simulink model "calefaccion_control_prueba_MODIFICADO_Jesus"  (R2021a)
settings: Solver=VariableStepAuto  StartTime=0.0  StopTime=3600*24*15  RelTol=1e-3
values from neighbouring files (symbols this model uses):
  Tref = 16.5    [izaro.m]
libraries: pid_lib x1
settings Model: Creator=izaro.garro  LastModifiedBy=djoroya
settings SolverCC: AlgebraicLoopSolver=TrustRegion
settings DebuggingCC: SFMachineParentedDataDiag=warning
settings SFSimCC: CustomCodeUndefinedFunction=UseInterfaceOnly

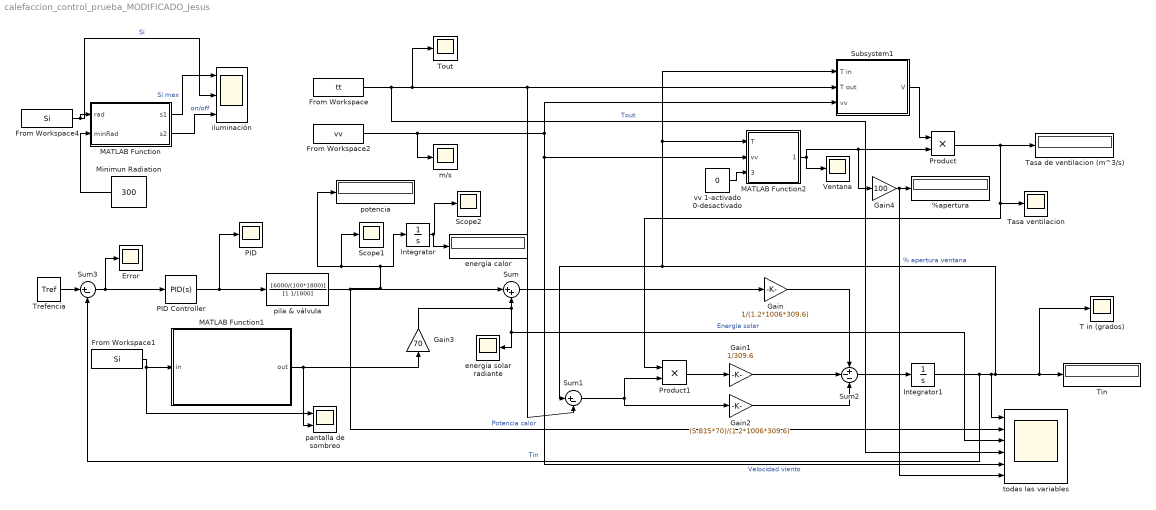
== system calefaccion_control_prueba_MODIFICADO_Jesus ==
  %apertura : Display
  Error : Scope
  From Workspace : FromWorkspace  VariableName=tt  SampleTime=600  ZeroCross=off
  From Workspace1 : FromWorkspace  VariableName=Si  SampleTime=600  ZeroCross=off
  From Workspace2 : FromWorkspace  VariableName=vv  SampleTime=600  ZeroCross=off
  From Workspace4 : FromWorkspace  VariableName=Si  SampleTime=600  ZeroCross=off
  Gain : Gain  Gain=1/(1.2*1006*309.6)
  Gain1 : Gain  Gain=1/309.6
  Gain2 : Gain  Gain=(5.815*70)/(1.2*1006*309.6)
  Gain3 : Gain  Gain=70
  Gain4 : Gain  Gain=100
  Integrator : Integrator
  Integrator1 : Integrator  InitialCondition=20
  MATLAB Function : MATLAB Function  TreatAsAtomicUnit=on  SystemSampleTime=600
  MATLAB Function1 : MATLAB Function  TreatAsAtomicUnit=on  SystemSampleTime=600
  MATLAB Function2 : MATLAB Function  TreatAsAtomicUnit=on  SystemSampleTime=1
  Minimun Radiation : Constant  Value=300
  PID : Scope
  PID Controller : pid_lib/PID Controller  Controller=PID  Form=Parallel  TimeDomain=Continuous-time  UseExternalTs=off  SampleTime=-1  IntegratorMethod=Forward Euler  FilterMethod=Forward Euler  ControllerParametersSource=internal  P=2  I=2/1200  D=0  UseFilter=on  N=0.0006  TunerSelectOption=Transfer Function Based (PID Tuner App)  ZeroCross=off  InitialConditionSource=internal  InitialConditionForIntegrator=0  InitialConditionForFilter=0  DifferentiatorICPrevScaledInput=0  ExternalReset=none  TrackingMode=off  Kt=1  LimitOutput=on  SatLimitsSource=internal  UpperSaturationLimit=100  LowerSaturationLimit=0  LinearizeAsGain=on  AntiWindupMode=clamping  Kb=1  POutMin=[]  POutMax=[]  IOutMin=[]  IOutMax=[]  DOutMin=[]  DOutMax=[]  NOutMin=[]  NOutMax=[]  SumOutMin=[]  SumOutMax=[]  SaturationOutMin=[]  SaturationOutMax=[]  PParamMin=[]  PParamMax=[]  IParamMin=[]  IParamMax=[]  DParamMin=[]  DParamMax=[]  NParamMin=[]  NParamMax=[]  KbParamMin=[]  KbParamMax=[]  KtParamMin=[]  KtParamMax=[]  KbOutMin=[]  KbOutMax=[]  KtOutMin=[]  KtOutMax=[]  IntegratorOutMin=[]  IntegratorOutMax=[]  FilterOutMin=[]  FilterOutMax=[]  SumI1OutMin=[]  SumI1OutMax=[]  SumI2OutMin=[]  SumI2OutMax=[]  SumI3OutMin=[]  SumI3OutMax=[]  SumI4OutMin=[]  SumI4OutMax=[]  SumDOutMin=[]  SumDOutMax=[]  DifferentiatorOutMin=[]  DifferentiatorOutMax=[]  FilterDiffOutCoefMin=[]  FilterDiffOutCoefMax=[]  ReciprocalOutMin=[]  ReciprocalOutMax=[]  SumDenOutMin=[]  SumDenOutMax=[]  SumNumOutMin=[]  SumNumOutMax=[]  DivideOutMin=[]  DivideOutMax=[]  UdiffTsProdOutMin=[]  UdiffTsProdOutMax=[]  NTsProdOutMin=[]  NTsProdOutMax=[]  UintegralTsProdOutMin=[]  UintegralTsProdOutMax=[]  UngainTsProdOutMin=[]  UngainTsProdOutMax=[]  IntegratorContinuousStateAttributes=''  IntegratorStateMustResolveToSignalObject=off  IntegratorRTWStateStorageClass=Auto  FilterContinuousStateAttributes=''  FilterStateMustResolveToSignalObject=off  FilterRTWStateStorageClass=Auto  ParallelPVariant=InternalParameters  IdealPVariant=Disabled  IVariant=InternalParameters  DVariant=InternalParameters  IntegratorVariant=Continuous  SatVariant=Enabled  AWVariant=ContClampingParallel  PCopyVariant=Disabled  TRVariant=Disabled  FdbkBlocksVariant=Forward  IdealPFdbkVariant=Disabled  SatFdbkVariant=Disabled  DerivativeFilterVariant=ContFilter  NVariant=InternalParameters  NCopyVariant=Disabled  FilterICVariant=InternalICsFilter  IntegratorICVariant=InternalICs  ExternalResetVariant=Disabled  TRSumVariant=Passthrough  SumFdbkVariant=Disabled  SumVariant=Sum_PID  TsampFilterVariant=InternalTs  TsampNgainVariant=Passthrough  TsampIntegralVariant=Passthrough  ExternalSaturationOutDataTypeStr=Inherit: Same as second input
  Product : Product
  Product1 : Product
  Scope1 : Scope
  Scope2 : Scope
  Subsystem1 : Subsystem
      mask Display: image('$imagefile'); % Use "Edit Image" on toolstrip to change.
  Sum : Sum  Inputs=|++
  Sum1 : Sum  Inputs=|+-
  Sum2 : Sum  Inputs=+--
  Sum3 : Sum  Inputs=|+-
  T in (grados) : Scope
  Tasa de ventilacion (m^3/s) : Display
  Tasa ventilacion : Scope
  Tin : Display
  Tout : Scope
  Trefencia : Constant  Value=Tref
  Ventana : Scope
  energía calor : Display
  energía solar radiante : Scope
  iluminación : Scope  NumInputPorts=3
  m/s : Scope
  pantalla de sombreo : Scope  NumInputPorts=2
  pila & válvula : TransferFcn  Numerator=[6000/(100*1800)]  Denominator=[1 1/1800]
  potencia : Display
  todas las variables : Scope  NumInputPorts=6
  vv 1-activado 0-desactivado : Constant  Value=0
  wires:
  Sum/1 -> Gain/1
  Gain/1 -> Sum2/1
  Gain1/1 -> Sum2/2
  Product1/1 -> Gain1/1
  Sum1/1 -> Gain2/1, Product1/2
  Gain2/1 -> Sum2/3
  Subsystem1/1(V) -> Product/1
  Sum3/1 -> Error/1, PID Controller/1
  PID Controller/1 -> PID/1, pila & válvula/1
  Trefencia/1 -> Sum3/1
  From Workspace/1 -> todas las variables/4, Tout/1, Sum1/2, Subsystem1/2(T out)  "Tout"
  pila & válvula/1 -> todas las variables/2, Sum/1, Integrator/1, potencia/1, Scope1/1  "Potencia calor"
  Integrator1/1 -> Sum3/2, todas las variables/1, T in (grados)/1, Tin/1, Sum1/1, MATLAB Function2/1(T), Subsystem1/1(T in)  "Tin"
  Gain3/1 -> todas las variables/3, energía solar radiante/1, Sum/2  "Energía solar"
  From Workspace4/1 -> iluminación/2, MATLAB Function/1(rad)  "Si"
  MATLAB Function/1(s1) -> iluminación/1  "Si max"
  MATLAB Function/2(s2) -> iluminación/3  "on/off"
  From Workspace2/1 -> Subsystem1/3(vv), todas las variables/5, MATLAB Function2/2(vv), m/s/1  "Velocidad viento"
  MATLAB Function1/1(out) -> Gain3/1, pantalla de sombreo/2
  From Workspace1/1 -> MATLAB Function1/1(in), pantalla de sombreo/1
  Product/1 -> Tasa de ventilacion (m^3/s)/1, Tasa ventilacion/1, Product1/1
  MATLAB Function2/1(posicionNueva) -> Ventana/1, Gain4/1, Product/2
  Gain4/1 -> todas las variables/6, %apertura/1  "% apertura ventana"
  vv 1-activado 0-desactivado/1 -> MATLAB Function2/3(vv_opcion)
  Integrator/1 -> Scope2/1, energía calor/1
  Sum2/1 -> Integrator1/1
  Minimun Radiation/1 -> MATLAB Function/2(minRad)

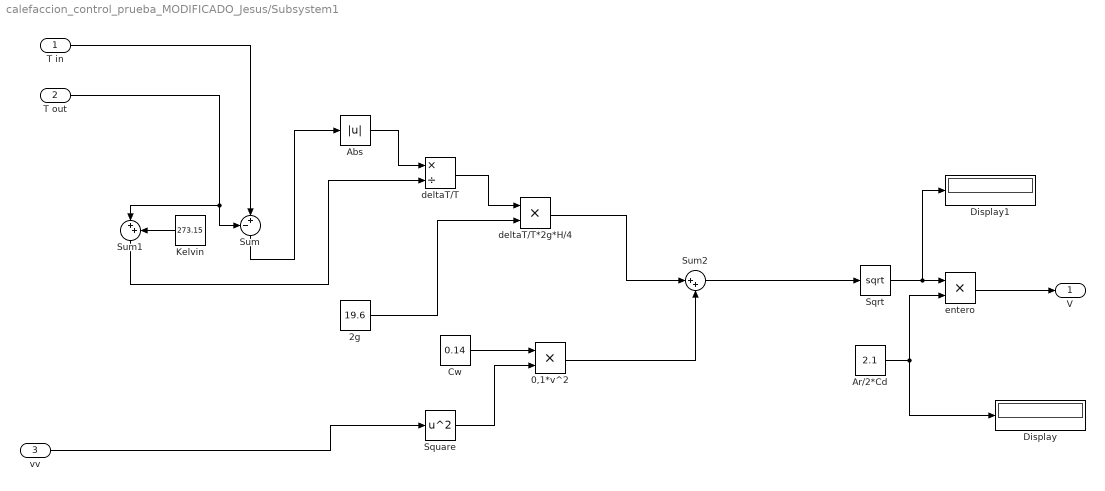
== system calefaccion_control_prueba_MODIFICADO_Jesus/Subsystem1 ==
  T in : Inport
  T out : Inport  Port=2
  vv : Inport  Port=3
  0,1*v^2 : Product  Inputs=**
  2g : Constant  Value=19.6
  Abs : Abs
  Ar/2*Cd : Constant  Value=2.1
  Cw : Constant  Value=0.14
  Display : Display
  Display1 : Display
  Kelvin : Constant  Value=273.15
  Sqrt : Sqrt  SaturateOnIntegerOverflow=on
  Square : Math  Operator=square  SignedPower=on  SaturateOnIntegerOverflow=on
  Sum : Sum  Inputs=-+|
  Sum1 : Sum  Inputs=|++
  Sum2 : Sum  Inputs=|++
  deltaT/T : Product  Inputs=*/
  deltaT/T*2g*H/4 : Product  Inputs=**
  entero : Product  Inputs=**
  V : Outport
  wires:
  T in/1 -> Sum/2
  Sum2/1 -> Sqrt/1
  Square/1 -> 0,1*v^2/2
  Cw/1 -> 0,1*v^2/1
  deltaT/T/1 -> deltaT/T*2g*H/4/1
  Sum1/1 -> deltaT/T/2
  Kelvin/1 -> Sum1/2
  T out/1 -> Sum1/1, Sum/1
  Ar/2*Cd/1 -> Display/1, entero/2
  deltaT/T*2g*H/4/1 -> Sum2/1
  2g/1 -> deltaT/T*2g*H/4/2
  0,1*v^2/1 -> Sum2/2
  Sqrt/1 -> Display1/1, entero/1
  entero/1 -> V/1
  vv/1 -> Square/1
  Abs/1 -> deltaT/T/1
  Sum/1 -> Abs/1

== matlab function calefaccion_control_prueba_MODIFICADO_Jesus/MATLAB Function1 ==
  settings: updateMethod=DISCRETE
  data: in input; out output
function out = pantallasombreo(in)

persistent flag;

if isempty(flag)
    flag = 0;
end

if in<15
    out=0;
    flag=0;
    
elseif in<=250
    out=in*0.95;
    flag=0;
elseif in>=300
    out=in*0.5;
    flag=1;
else
    if flag==1
        out=in*0.5;
    else
        out=in*0.95;
    end
end

== matlab function calefaccion_control_prueba_MODIFICADO_Jesus/MATLAB Function ==
  settings: updateMethod=DISCRETE
  data: rad input; s1 output; s2 output; minRad input
function [s1,s2]=radmax(rad,minRad)

persistent max;
persistent aux;

if isempty(max)
    max = 0;
end

if isempty(aux)
    aux = 0;
end

%%
aux=aux+1;

if aux<145 
    if (rad>max)
        max=rad;
    end
else
    aux=0;
    max=0;
end

% minRad = 185.19; Izaro

if aux<115 || aux>133
    s2=0;
else
    if (max<minRad)
        s2=1;
    else
        s2=0;
    end
end

s1=max;

end

== matlab function calefaccion_control_prueba_MODIFICADO_Jesus/MATLAB Function2 ==
  settings: updateMethod=DISCRETE
  data: T input; posicionNueva output; vv input; vv_opcion input
function posicionNueva  = ventanas(T,vv,vv_opcion)

persistent posicionAnterior;

if isempty(posicionAnterior)
    posicionAnterior = 0;
end


posicionIdeal = CalcularPosicion(T, 20);

if abs(posicionIdeal - posicionAnterior) < 0.1
    posicionNueva = posicionAnterior;   
else
    if posicionIdeal > posicionAnterior
        posicionNueva = posicionAnterior + 0.1;
    else
        posicionNueva = posicionAnterior - 0.1;
    end
end

if vv_opcion==1
    if vv>10 && posicionNueva>0.3
        posicionNueva=0.3;
    end
end

posicionAnterior = posicionNueva;
end

function apertura= CalcularPosicion(temperatura, consigna)
if temperatura > consigna
    apertura = (temperatura - consigna) / 10;
    if apertura > 1
        apertura = 1;
    end
else
    apertura = 0;
end
end
